simulink model "Calibrating_The_AR_Drone_Camera_Model"  (R2016a)
settings: configuration reference "AR_Drone_ConfigSet" (kept outside this file)
libraries: AR_Drone_Video x1, AR_Drone_Video_Processing x1
settings Model: DataDictionary=ArDroneDataDictionary.sldd  SimulationMode=external  Creator=sannem  LastModifiedBy=sannem
settings ConfigSetRef: DDName=ArDroneDataDictionary.sldd

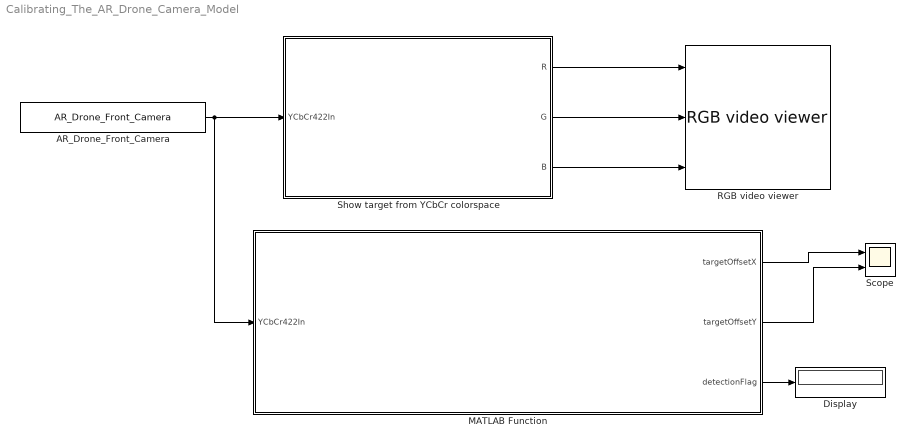
== system Calibrating_The_AR_Drone_Camera_Model ==
  AR_Drone_Front_Camera : AR_Drone_Video/AR_Drone_Front_Camera  SFunctionSpec=videoGrabImage1(uint8 y1[1843200])  SampleTime=0.1  ShowSpec=off
  Display : Display
  MATLAB Function : MATLAB Function  TreatAsAtomicUnit=on  mask(AR Drone:  Find Colored Object Position){width=1280, height=720, downScaleFactor=5, cbFloor=0, cbCeiling=117, crFloor=0, crCeiling=117, pixelThreshold=10}
      mask prompts: width "Video input width"; height "Video input height"; downScaleFactor "Video down sample factor"; cbFloor "Blue shift minimum [0-255]"; cbCeiling "Blue shift maximum [0-255]"; crFloor "Red shift minimum [0-255]"; crCeiling "Red shift maximum [0-255]"; pixelThreshold "Minimum object detection pixel count"
      mask help:
      | This MATLAB function block takes an input video stream, down samples in both the horizontal and veritcal direction to reduce the computational demand, and then determines how many pixels fall within the user specified colorspace region and what their average postition is in the video. If you are experiencing some artifacts which are hard to tune out, increase the minimum target pixel count. No target will be registered (detectionFlag = 0) unless as many pixels as you define are found in the target colorspace (detectionFlag = 1).
      | The output x and y position are scaled between -1 and 1.
      |
      | Using the YCbCr colorspace some recommend values are:
      |
      | Green target:
      | cb[min, max] = [0, 100]
      | cr[min, max] = [0, 100]
      |
      | Blue target:
      | cb[min, max] = [155, 255]
      | cr[min, max] = [0, 100]
      |
      | Red target:
      | cb[min, max] = [0, 100]
      | cr[min, max] = [155, 255]
  RGB video viewer : AR_Drone_Video_Processing/RGB video viewer
  Scope : Scope  NumInputPorts=2
  Show target from YCbCr colorspace : MATLAB Function  TreatAsAtomicUnit=on  mask(ARDrone: Find Target In YCbCr Colorspace){width=1280, height=720, downScaleFactor=5, cbFloor=0, cbCeiling=118, crFloor=0, crCeiling=118, pixelThreshold=10}
      mask prompts: width "Video input width"; height "Video input height"; downScaleFactor "Video downsample factor"; cbFloor "Blue shift minimum [0-255]"; cbCeiling "Blue shift maximum [0-255]"; crFloor "Red shift minimum [0-255]"; crCeiling "Red shift maximum [0-255]"; pixelThreshold "Minimum object detection pixel count"
      mask help:
      | This MATLAB function block takes an input video stream, down samples in both the horizontal and veritcal direction to reduce the computational demand, and then determines how many pixels fall within the user specified colorspace region and what their average postition is in the video. If you are experiencing some artifacts which are hard to tune out, increase the minimum target pixel count. No target will be registered unless as many pixels as you define are found in the target colorspace.
      |
      | Using the YCbCr colorspace some recommend values are:
      |
      | Green target:
      | cb[min, max] = [0, 100]
      | cr[min, max] = [0, 100]
      |
      | Blue target:
      | cb[min, max] = [155, 255]
      | cr[min, max] = [0, 100]
      |
      | Red target:
      | cb[min, max] = [0, 100]
      | cr[min, max] = [155, 255]
  wires:
  AR_Drone_Front_Camera/1 -> MATLAB Function/1(YCbCr422In), Show target from YCbCr colorspace/1(YCbCr422In)
  Show target from YCbCr colorspace/3(B) -> RGB video viewer/3
  Show target from YCbCr colorspace/2(G) -> RGB video viewer/2
  Show target from YCbCr colorspace/1(R) -> RGB video viewer/1
  MATLAB Function/1(targetOffsetX) -> Scope/1
  MATLAB Function/2(targetOffsetY) -> Scope/2
  MATLAB Function/3(detectionFlag) -> Display/1

== matlab function Calibrating_The_AR_Drone_Camera_Model/MATLAB Function ==
  data: YCbCr422In input; targetOffsetX output; targetOffsetY output; detectionFlag output; cbFloor parameter; cbCeiling parameter; crFloor parameter; crCeiling parameter; downScaleFactor parameter; height parameter; width parameter; pixelThreshold parameter
function [targetOffsetX, targetOffsetY, detectionFlag]  = coloredObjectPosition(YCbCr422In,cbFloor, cbCeiling, crFloor, crCeiling, downScaleFactor, height, width, pixelThreshold)

xPositionSum = 0;
yPositionSum = 0;
targetOffsetX = 0;
targetOffsetY = 0;
targetPixelCount = 0;
detectionFlag = 0;

for verticalIndex = 1 : 1 : height/downScaleFactor;             % indexing for downsampled vertical direction
    for horizontalIndex = 1 : 1 : (width / 2)/downScaleFactor;  % indexing for downsampled horizontal direction
        index = 4 * (downScaleFactor * (verticalIndex - 1) * (width / 2) + downScaleFactor * horizontalIndex) - 3;  % translate the horizontal and vertical indexes into the index into the video input
        pixel = double([YCbCr422In(index) YCbCr422In(index+1) YCbCr422In(index+2) YCbCr422In(index+3)]);    % retrieve the pixel data and convert for calculation

        %% verify whether this pixel is within the user specified region of the YCbCr colorspace
        if ( pixel(1)  >= cbFloor && pixel(1)  <= cbCeiling && ...
             pixel(3)  >= crFloor && pixel(3)  <= crCeiling  )

            targetPixelCount = targetPixelCount + 1;
            xPositionSum = xPositionSum + 2 * horizontalIndex * downScaleFactor;
            yPositionSum = yPositionSum + verticalIndex * downScaleFactor;
        end
    end
end

% compute the average green pixel position
if targetPixelCount > pixelThreshold
    detectionFlag = 1;
    targetOffsetX = xPositionSum / targetPixelCount / (0.5 * width) - 1;     
    targetOffsetY = -(yPositionSum / targetPixelCount / (0.5 * height) - 1);
else
    % not enough pixels were target pixels:

end

end

== matlab function Calibrating_The_AR_Drone_Camera_Model/Show target from YCbCr colorspace ==
  data: YCbCr422In input; cbFloor parameter; cbCeiling parameter; crFloor parameter; crCeiling parameter; downScaleFactor parameter; height parameter; width parameter; R output; G output; B output; pixelThreshold parameter
function [R, G, B]  = showYCbCrTarget(YCbCr422In,cbFloor, cbCeiling, crFloor, crCeiling, downScaleFactor, height, width, pixelThreshold)

xPositionSum = 0;
yPositionSum = 0;
xPositionMean = -1;
yPositionMean = -1;
targetPixelCount = 0;

%% create a 'RGB' matrix for showing the detected pixels
R = uint8(zeros((width / 2)/downScaleFactor, height/downScaleFactor));

for verticalIndex = 1 : 1 : height/downScaleFactor;             % indexing for downsampled vertical direction
    for horizontalIndex = 1 : 1 : (width / 2)/downScaleFactor;  % indexing for downsampled horizontal direction
        index = 4 * (downScaleFactor * (verticalIndex - 1) * (width / 2) + downScaleFactor * horizontalIndex) - 3;  % translate the horizontal and vertical indexes into the index into the video input
        pixel = double([YCbCr422In(index) YCbCr422In(index+1) YCbCr422In(index+2) YCbCr422In(index+3)]);    % retrieve the pixel data and convert for calculation

        %% verify whether this pixel is within the user specified region of the YCbCr colorspace
        if ( pixel(1)  >= cbFloor && pixel(1)  <= cbCeiling && ...
             pixel(3)  >= crFloor && pixel(3)  <= crCeiling  )

            targetPixelCount = targetPixelCount + 1;
            xPositionSum = xPositionSum + horizontalIndex * downScaleFactor;
            yPositionSum = yPositionSum + verticalIndex * downScaleFactor;
            % set the targetView
            R(horizontalIndex,verticalIndex) = uint8(255);

        end
    end
end

% compute the average green pixel position
if targetPixelCount > pixelThreshold
    % copy the target view to B and G such it becomes white
    B = R;
    G = R;
    xPositionMean = xPositionSum / targetPixelCount;     
    yPositionMean = yPositionSum / targetPixelCount;
    % mark this position as a red pixel
    xScale = xPositionMean / downScaleFactor;
    yScale = yPositionMean / downScaleFactor;
    R(floor(xScale),floor(yScale)) = uint8(255);
    G(floor(xScale),floor(yScale)) = 0;
    B(floor(xScale),floor(yScale)) = 0;
else
    % not enough pixels were target pixels so reset R
    R = uint8(zeros((width / 2)/downScaleFactor, height/downScaleFactor));
    B = R;
    G = R;
end

end
